simulink model "HITL_DEMO_2"  (R2022a)
settings: Solver=FixedStepAuto  StartTime=0.0  StopTime=100  FixedStep=.001  MaxStep=0.01  RelTol=1e-3
libraries: etargetslib x2, instrumentlib x1
settings Model: Creator=kiran  LastModifiedBy=usmaanyaqoob
settings SolverCC: AutoInsertRateTranBlk=on
settings DebuggingCC: UnconnectedInputMsg=warning  UnconnectedOutputMsg=warning  UnconnectedLineMsg=warning
settings RTWCC: DLArmComputeVersion=19.05

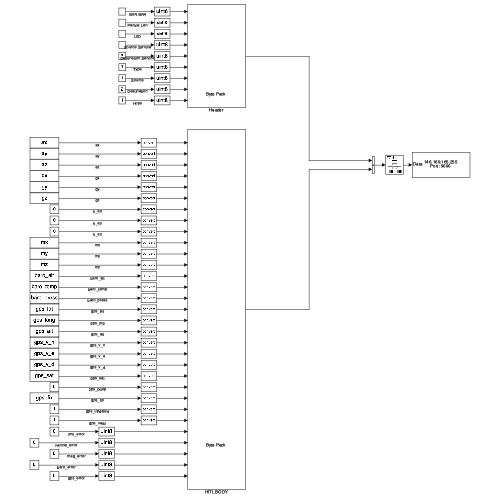
[thumbnail: Simulink's stored preview of the top-level diagram]
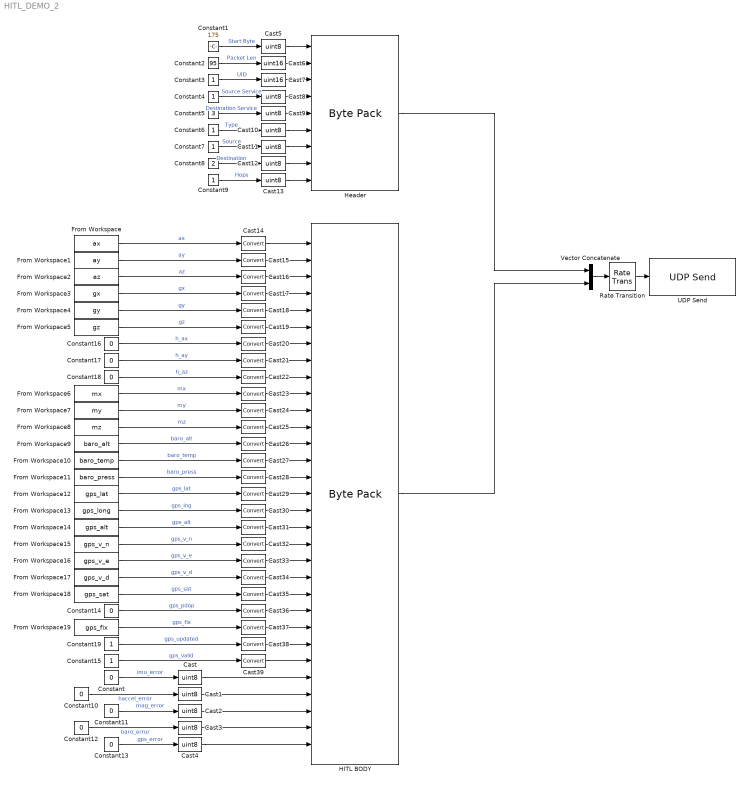
== system HITL_DEMO_2 ==
  Cast{,1..5,8..13} (12 alike) : DataTypeConversion  OutDataTypeStr=uint8  SaturateOnIntegerOverflow=off  RndMeth=Floor
  Cast{14..39} (26 alike) : DataTypeConversion  SaturateOnIntegerOverflow=off  RndMeth=Floor
  Cast6 : DataTypeConversion  OutDataTypeStr=uint16  SaturateOnIntegerOverflow=off  RndMeth=Floor
  Cast7 : DataTypeConversion  OutDataTypeStr=uint16  SaturateOnIntegerOverflow=off  RndMeth=Floor
  Constant{,10..14,16..18} (9 alike) : Constant  Value=0
  Constant1 : Constant  Value=175
  Constant{3..4,6..7,9,15,19} (7 alike) : Constant
  Constant2 : Constant  Value=95
  Constant5 : Constant  Value=3
  Constant8 : Constant  Value=2
  From Workspace : FromWorkspace  VariableName=ax  OutputAfterFinalValue=Setting to zero
  From Workspace1 : FromWorkspace  VariableName=ay  OutputAfterFinalValue=Setting to zero
  From Workspace10 : FromWorkspace  VariableName=baro_temp  OutputAfterFinalValue=Setting to zero
  From Workspace11 : FromWorkspace  VariableName=baro_press  OutputAfterFinalValue=Setting to zero
  From Workspace12 : FromWorkspace  VariableName=gps_lat  OutputAfterFinalValue=Setting to zero
  From Workspace13 : FromWorkspace  VariableName=gps_long  OutputAfterFinalValue=Setting to zero
  From Workspace14 : FromWorkspace  VariableName=gps_alt  OutputAfterFinalValue=Setting to zero
  From Workspace15 : FromWorkspace  VariableName=gps_v_n  OutputAfterFinalValue=Setting to zero
  From Workspace16 : FromWorkspace  VariableName=gps_v_e  OutputAfterFinalValue=Setting to zero
  From Workspace17 : FromWorkspace  VariableName=gps_v_d  OutputAfterFinalValue=Setting to zero
  From Workspace18 : FromWorkspace  VariableName=gps_sat  OutputAfterFinalValue=Setting to zero
  From Workspace19 : FromWorkspace  VariableName=gps_fix  OutputAfterFinalValue=Setting to zero
  From Workspace2 : FromWorkspace  VariableName=az  OutputAfterFinalValue=Setting to zero
  From Workspace3 : FromWorkspace  VariableName=gx  OutputAfterFinalValue=Setting to zero
  From Workspace4 : FromWorkspace  VariableName=gy  OutputAfterFinalValue=Setting to zero
  From Workspace5 : FromWorkspace  VariableName=gz  OutputAfterFinalValue=Setting to zero
  From Workspace6 : FromWorkspace  VariableName=mx  OutputAfterFinalValue=Setting to zero
  From Workspace7 : FromWorkspace  VariableName=my  OutputAfterFinalValue=Setting to zero
  From Workspace8 : FromWorkspace  VariableName=mz  OutputAfterFinalValue=Setting to zero
  From Workspace9 : FromWorkspace  VariableName=baro_alt  OutputAfterFinalValue=Setting to zero
  HITL BODY : etargetslib/Byte Pack  datatypes={'single','single','single','single','single','single','single','single','single','single','single','single','single','single','single','single','single','int32','int32','int32','int32','uint8','uint16','uint8','uint8','uint8','uint8','uint8','uint8','uint8','uint8'}  byteAlign=1
  Header : etargetslib/Byte Pack  datatypes={'uint8','uint16','uint16','uint8','uint8','uint8','uint8','uint8','uint8'}  byteAlign=1
  Rate Transition : RateTransition  OutPortSampleTime=.1
  UDP Send : instrumentlib/UDP Send  Host=146.169.165.255  Port=9090  LocalPort=-1  EnablePortSharing=off  ByteOrder=LittleEndian  OutputDatagramPacketSize=512  EnableBlockingMode=on  LocalAddress=0.0.0.0
  Vector Concatenate : Concatenate
  wires:
  Vector Concatenate/1 -> Rate Transition/1
  Header/1 -> Vector Concatenate/1
  HITL BODY/1 -> Vector Concatenate/2
  From Workspace/1 -> Cast14/1  "ax"
  From Workspace1/1 -> Cast15/1  "ay"
  From Workspace2/1 -> Cast16/1  "az"
  From Workspace3/1 -> Cast17/1  "gx"
  From Workspace5/1 -> Cast19/1  "gz"
  Constant16/1 -> Cast20/1  "h_ax"
  Constant17/1 -> Cast21/1  "h_ay"
  Constant18/1 -> Cast22/1  "h_az"
  From Workspace6/1 -> Cast23/1  "mx"
  From Workspace7/1 -> Cast24/1  "my"
  From Workspace8/1 -> Cast25/1  "mz"
  From Workspace9/1 -> Cast26/1  "baro_alt"
  From Workspace10/1 -> Cast27/1  "baro_temp"
  From Workspace11/1 -> Cast28/1  "baro_press"
  From Workspace12/1 -> Cast29/1  "gps_lat"
  From Workspace13/1 -> Cast30/1  "gps_lng"
  From Workspace14/1 -> Cast31/1  "gps_alt"
  From Workspace15/1 -> Cast32/1  "gps_v_n"
  From Workspace16/1 -> Cast33/1  "gps_v_e"
  From Workspace17/1 -> Cast34/1  "gps_v_d"
  From Workspace18/1 -> Cast35/1  "gps_sat"
  Constant14/1 -> Cast36/1  "gps_pdop"
  From Workspace19/1 -> Cast37/1  "gps_fix"
  Constant19/1 -> Cast38/1  "gps_updated"
  Constant15/1 -> Cast39/1  "gps_valid"
  From Workspace4/1 -> Cast18/1  "gy"
  Constant1/1 -> Cast5/1  "Start Byte"
  Constant2/1 -> Cast6/1  "Packet Len"
  Constant3/1 -> Cast7/1  "UID"
  Constant4/1 -> Cast8/1  "Source Service"
  Constant5/1 -> Cast9/1  "Destination Service"
  Constant6/1 -> Cast10/1  "Type"
  Constant7/1 -> Cast11/1  "Source"
  Constant8/1 -> Cast12/1  "Destination"
  Constant9/1 -> Cast13/1  "Hops"
  Cast2/1 -> HITL BODY/29
  Cast3/1 -> HITL BODY/30
  Cast4/1 -> HITL BODY/31
  Cast5/1 -> Header/1
  Cast6/1 -> Header/2
  Cast7/1 -> Header/3
  Cast8/1 -> Header/4
  Cast9/1 -> Header/5
  Cast10/1 -> Header/6
  Cast11/1 -> Header/7
  Cast12/1 -> Header/8
  Cast13/1 -> Header/9
  Cast14/1 -> HITL BODY/1
  Cast15/1 -> HITL BODY/2
  Cast16/1 -> HITL BODY/3
  Cast17/1 -> HITL BODY/4
  Cast18/1 -> HITL BODY/5
  Cast19/1 -> HITL BODY/6
  Cast20/1 -> HITL BODY/7
  Cast25/1 -> HITL BODY/12
  Cast23/1 -> HITL BODY/10
  Cast27/1 -> HITL BODY/14
  Cast26/1 -> HITL BODY/13
  Cast22/1 -> HITL BODY/9
  Cast24/1 -> HITL BODY/11
  Cast21/1 -> HITL BODY/8
  Cast39/1 -> HITL BODY/26
  Cast/1 -> HITL BODY/27
  Cast1/1 -> HITL BODY/28
  Cast36/1 -> HITL BODY/23
  Cast38/1 -> HITL BODY/25
  Cast37/1 -> HITL BODY/24
  Cast35/1 -> HITL BODY/22
  Cast33/1 -> HITL BODY/20
  Cast32/1 -> HITL BODY/19
  Cast34/1 -> HITL BODY/21
  Cast31/1 -> HITL BODY/18
  Cast28/1 -> HITL BODY/15
  Cast30/1 -> HITL BODY/17
  Cast29/1 -> HITL BODY/16
  Rate Transition/1 -> UDP Send/1
  Constant10/1 -> Cast1/1  "haccel_error"
  Constant13/1 -> Cast4/1  "gps_error"
  Constant12/1 -> Cast3/1  "baro_error"
  Constant11/1 -> Cast2/1  "mag_error"
  Constant/1 -> Cast/1  "imu_error"
